simulink library "INT_EngBrk_ExhFlpCtl"  (R2016b)
settings: Solver=VariableStepAuto  StartTime=0.0  StopTime=10.0  RelTol=1e-3
settings Model: Creator=lenovo  LastModifiedBy=lenovo

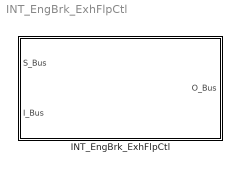
== system INT_EngBrk_ExhFlpCtl ==
  INT_EngBrk_ExhFlpCtl : Subsystem

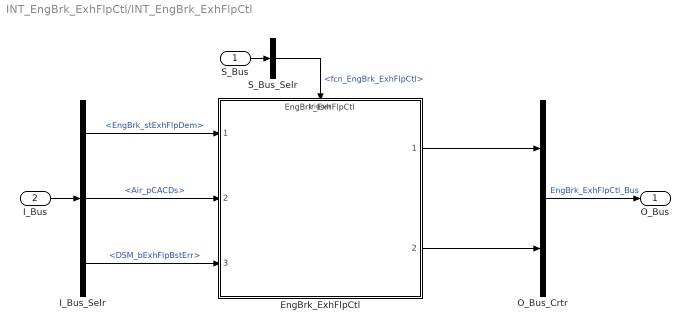
== system INT_EngBrk_ExhFlpCtl/INT_EngBrk_ExhFlpCtl ==
  S_Bus : Inport
  I_Bus : Inport  Port=2
  EngBrk_ExhFlpCtl : ModelReference  ModelNameDialog=EngBrk_ExhFlpCtl  ModelReferenceVersion=1.2  TriggerPortName=function  TriggerPortTriggerType=function-call  TriggerPortStatesWhenEnabling=held
  I_Bus_Selr : BusSelector  OutputSignals=EngBrk_stExhFlpDem,Air_pCACDs,DSM_bExhFlpBstErr
  O_Bus_Crtr : BusCreator  Inputs=2
  S_Bus_Selr : BusSelector  OutputSignals=fcn_EngBrk_ExhFlpCtl
  O_Bus : Outport
  wires:
  S_Bus_Selr/1 -> EngBrk_ExhFlpCtl/Trigger  "<fcn_EngBrk_ExhFlpCtl>"
  S_Bus/1 -> S_Bus_Selr/1
  I_Bus/1 -> I_Bus_Selr/1
  I_Bus_Selr/1 -> EngBrk_ExhFlpCtl/1  "<EngBrk_stExhFlpDem>"
  I_Bus_Selr/2 -> EngBrk_ExhFlpCtl/2  "<Air_pCACDs>"
  I_Bus_Selr/3 -> EngBrk_ExhFlpCtl/3  "<DSM_bExhFlpBstErr>"
  O_Bus_Crtr/1 -> O_Bus/1  "EngBrk_ExhFlpCtl_Bus"
  EngBrk_ExhFlpCtl/1 -> O_Bus_Crtr/1
  EngBrk_ExhFlpCtl/2 -> O_Bus_Crtr/2
